simulink library "tramontina_database_nvidialib"  (R2023b)
settings: Solver=VariableStepAuto  StartTime=0.0  StopTime=10.0  RelTol=1e-3
libraries: canmsglib x26, simulink x1
settings Model: Creator=matlab.cut  LastModifiedBy=matlab.cut

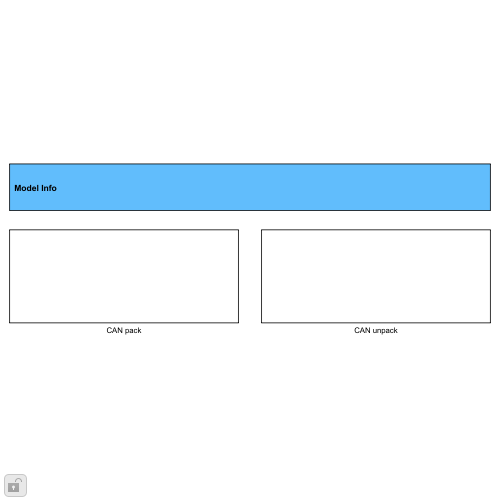
[thumbnail: Simulink's stored preview of the top-level diagram]
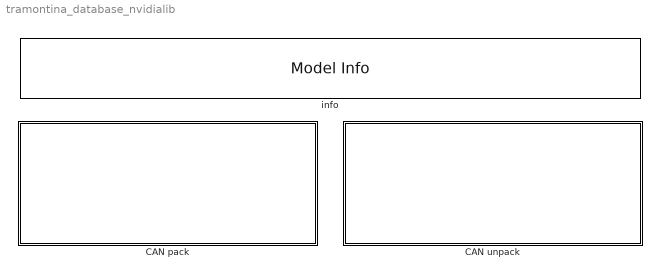
== system tramontina_database_nvidialib ==
  CAN pack : Subsystem
  CAN unpack : Subsystem
  info : simulink/Model-Wide Utilities/Model Info  Frame=on  DisplayStringWithTags=SPEEDGOAT CAN Database Library for: tramontina_database_nvidia  HorizontalTextAlignment=Left  LeftAlignmentValue=0.01

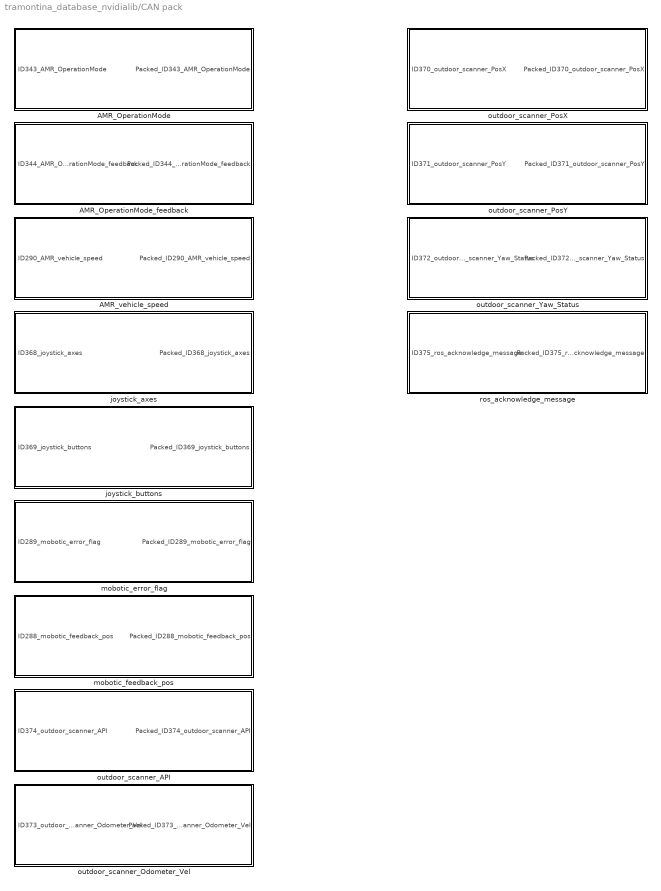
== system tramontina_database_nvidialib/CAN pack ==
  AMR_OperationMode : Subsystem
  AMR_OperationMode_feedback : Subsystem
  AMR_vehicle_speed : Subsystem
  joystick_axes : Subsystem
  joystick_buttons : Subsystem
  mobotic_error_flag : Subsystem
  mobotic_feedback_pos : Subsystem
  outdoor_scanner_API : Subsystem
  outdoor_scanner_Odometer_Vel : Subsystem
  outdoor_scanner_PosX : Subsystem
  outdoor_scanner_PosY : Subsystem
  outdoor_scanner_Yaw_Status : Subsystem
  ros_acknowledge_message : Subsystem

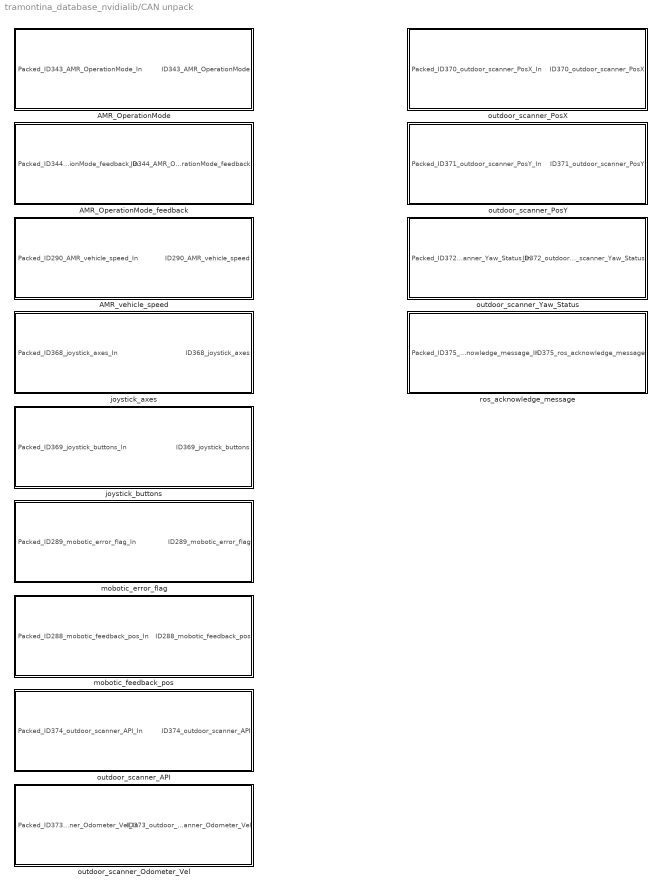
== system tramontina_database_nvidialib/CAN unpack ==
  AMR_OperationMode : Subsystem
  AMR_OperationMode_feedback : Subsystem
  AMR_vehicle_speed : Subsystem
  joystick_axes : Subsystem
  joystick_buttons : Subsystem
  mobotic_error_flag : Subsystem
  mobotic_feedback_pos : Subsystem
  outdoor_scanner_API : Subsystem
  outdoor_scanner_Odometer_Vel : Subsystem
  outdoor_scanner_PosX : Subsystem
  outdoor_scanner_PosY : Subsystem
  outdoor_scanner_Yaw_Status : Subsystem
  ros_acknowledge_message : Subsystem

== system tramontina_database_nvidialib/CAN pack/AMR_OperationMode ==
  In Bus Element : Inport  PortName=ID343_AMR_OperationMode  Element=OperationMode
  AMR_OperationMode : canmsglib/CAN Pack  CANdbFile=C:\Users\matlab.cut\Desktop\AMR\canbus_files\tramontina_database_nvidia.dbc  MsgList=AMR_OperationMode  MsgName=AMR_OperationMode  MsgIDType=Standard (11-bit identifier)  MsgIdentifier=343  MsgLength=8  Remote=off  ApplyMinMax=off  BusOutput=on  SignalInfo={'OperationMode','0','3','LE','unsigned','Standard','0','1','0','-Inf','Inf'}
      settings: DataFormat=manually specified signals
  Packed_ID343_AMR_OperationMode : Outport
  wires:
  AMR_OperationMode/1 -> Packed_ID343_AMR_OperationMode/1
  In Bus Element/1 -> AMR_OperationMode/1

== system tramontina_database_nvidialib/CAN pack/AMR_OperationMode_feedback ==
  In Bus Element : Inport  PortName=ID344_AMR_OperationMode_feedback  Element=OperationMode_auto
  In Bus Element1 : Inport  PortName=ID344_AMR_OperationMode_feedback  Element=OperationMode_idle
  In Bus Element2 : Inport  PortName=ID344_AMR_OperationMode_feedback  Element=OperationMode_manual
  AMR_OperationMode_feedback : canmsglib/CAN Pack  CANdbFile=C:\Users\matlab.cut\Desktop\AMR\canbus_files\tramontina_database_nvidia.dbc  MsgList=AMR_OperationMode_feedback  MsgName=AMR_OperationMode_feedback  MsgIDType=Standard (11-bit identifier)  MsgIdentifier=344  MsgLength=8  Remote=off  ApplyMinMax=off  BusOutput=on  SignalInfo={'OperationMode_auto','2','1','LE','unsigned','Standard','0','1','0','-Inf','Inf';'OperationMode_idle','0','1','LE','unsigned','Standard','0','1','0','-Inf','Inf';'OperationMode_manual','1','1','LE','unsigned','Standard','0','1','0','-Inf','Inf'}
      settings: DataFormat=manually specified signals
  Packed_ID344_AMR_OperationMode_feedback : Outport
  wires:
  AMR_OperationMode_feedback/1 -> Packed_ID344_AMR_OperationMode_feedback/1
  In Bus Element/1 -> AMR_OperationMode_feedback/1
  In Bus Element1/1 -> AMR_OperationMode_feedback/2
  In Bus Element2/1 -> AMR_OperationMode_feedback/3

== system tramontina_database_nvidialib/CAN pack/AMR_vehicle_speed ==
  In Bus Element : Inport  PortName=ID290_AMR_vehicle_speed  Element=speed_m_per_min
  In Bus Element1 : Inport  PortName=ID290_AMR_vehicle_speed  Element=speed_m_per_s
  AMR_vehicle_speed : canmsglib/CAN Pack  CANdbFile=C:\Users\matlab.cut\Desktop\AMR\canbus_files\tramontina_database_nvidia.dbc  MsgList=AMR_vehicle_speed  MsgName=AMR_vehicle_speed  MsgIDType=Standard (11-bit identifier)  MsgIdentifier=290  MsgLength=8  Remote=off  ApplyMinMax=off  BusOutput=on  SignalInfo={'speed_m_per_min','0','32','LE','single','Standard','0','1','0','-90','90';'speed_m_per_s','32','32','LE','single','Standard','0','1','0','-1.5','1.5'}
      settings: DataFormat=manually specified signals
  Packed_ID290_AMR_vehicle_speed : Outport
  wires:
  AMR_vehicle_speed/1 -> Packed_ID290_AMR_vehicle_speed/1
  In Bus Element/1 -> AMR_vehicle_speed/1
  In Bus Element1/1 -> AMR_vehicle_speed/2

== system tramontina_database_nvidialib/CAN pack/joystick_axes ==
  In Bus Element : Inport  PortName=ID368_joystick_axes  Element=joystick_direction
  In Bus Element1 : Inport  PortName=ID368_joystick_axes  Element=joystick_throttle
  joystick_axes : canmsglib/CAN Pack  CANdbFile=C:\Users\matlab.cut\Desktop\AMR\canbus_files\tramontina_database_nvidia.dbc  MsgList=joystick_axes  MsgName=joystick_axes  MsgIDType=Standard (11-bit identifier)  MsgIdentifier=368  MsgLength=8  Remote=off  ApplyMinMax=off  BusOutput=on  SignalInfo={'joystick_direction','56','32','BE','single','Standard','0','1','0','-1','1';'joystick_throttle','24','32','BE','single','Standard','0','1','0','-1','1'}
      settings: DataFormat=manually specified signals
  Packed_ID368_joystick_axes : Outport
  wires:
  joystick_axes/1 -> Packed_ID368_joystick_axes/1
  In Bus Element/1 -> joystick_axes/1
  In Bus Element1/1 -> joystick_axes/2

== system tramontina_database_nvidialib/CAN pack/joystick_buttons ==
  In Bus Element : Inport  PortName=ID369_joystick_buttons  Element=button_5
  In Bus Element1 : Inport  PortName=ID369_joystick_buttons  Element=button_6
  joystick_buttons : canmsglib/CAN Pack  CANdbFile=C:\Users\matlab.cut\Desktop\AMR\canbus_files\tramontina_database_nvidia.dbc  MsgList=joystick_buttons  MsgName=joystick_buttons  MsgIDType=Standard (11-bit identifier)  MsgIdentifier=369  MsgLength=1  Remote=off  ApplyMinMax=off  BusOutput=on  SignalInfo={'button_5','4','1','LE','unsigned','Standard','0','1','0','-Inf','Inf';'button_6','5','1','LE','unsigned','Standard','0','1','0','-Inf','Inf'}
      settings: DataFormat=manually specified signals
  Packed_ID369_joystick_buttons : Outport
  wires:
  joystick_buttons/1 -> Packed_ID369_joystick_buttons/1
  In Bus Element/1 -> joystick_buttons/1
  In Bus Element1/1 -> joystick_buttons/2

== system tramontina_database_nvidialib/CAN pack/mobotic_error_flag ==
  In Bus Element : Inport  PortName=ID289_mobotic_error_flag  Element=steering_unit_error
  mobotic_error_flag : canmsglib/CAN Pack  CANdbFile=C:\Users\matlab.cut\Desktop\AMR\canbus_files\tramontina_database_nvidia.dbc  MsgList=mobotic_error_flag  MsgName=mobotic_error_flag  MsgIDType=Standard (11-bit identifier)  MsgIdentifier=289  MsgLength=8  Remote=off  ApplyMinMax=off  BusOutput=on  SignalInfo={'steering_unit_error','0','1','LE','unsigned','Standard','0','1','0','-Inf','Inf'}
      settings: DataFormat=manually specified signals
  Packed_ID289_mobotic_error_flag : Outport
  wires:
  mobotic_error_flag/1 -> Packed_ID289_mobotic_error_flag/1
  In Bus Element/1 -> mobotic_error_flag/1

== system tramontina_database_nvidialib/CAN pack/mobotic_feedback_pos ==
  In Bus Element : Inport  PortName=ID288_mobotic_feedback_pos  Element=enconder_feedback
  In Bus Element1 : Inport  PortName=ID288_mobotic_feedback_pos  Element=position_feedback
  mobotic_feedback_pos : canmsglib/CAN Pack  CANdbFile=C:\Users\matlab.cut\Desktop\AMR\canbus_files\tramontina_database_nvidia.dbc  MsgList=mobotic_feedback_pos  MsgName=mobotic_feedback_pos  MsgIDType=Standard (11-bit identifier)  MsgIdentifier=288  MsgLength=8  Remote=off  ApplyMinMax=off  BusOutput=on  SignalInfo={'enconder_feedback','32','32','LE','signed','Standard','0','1','0','-Inf','Inf';'position_feedback','0','32','LE','signed','Standard','0','0.087891','30','-75','75'}
      settings: DataFormat=manually specified signals
  Packed_ID288_mobotic_feedback_pos : Outport
  wires:
  mobotic_feedback_pos/1 -> Packed_ID288_mobotic_feedback_pos/1
  In Bus Element/1 -> mobotic_feedback_pos/1
  In Bus Element1/1 -> mobotic_feedback_pos/2

== system tramontina_database_nvidialib/CAN pack/outdoor_scanner_API ==
  In Bus Element : Inport  PortName=ID374_outdoor_scanner_API  Element=LocClearMap
  In Bus Element1 : Inport  PortName=ID374_outdoor_scanner_API  Element=LocInitAtPose
  In Bus Element2 : Inport  PortName=ID374_outdoor_scanner_API  Element=LocLoadMap
  In Bus Element3 : Inport  PortName=ID374_outdoor_scanner_API  Element=LocSetMap
  In Bus Element4 : Inport  PortName=ID374_outdoor_scanner_API  Element=MapID
  outdoor_scanner_API : canmsglib/CAN Pack  CANdbFile=C:\Users\matlab.cut\Desktop\AMR\canbus_files\tramontina_database_nvidia.dbc  MsgList=outdoor_scanner_API  MsgName=outdoor_scanner_API  MsgIDType=Standard (11-bit identifier)  MsgIdentifier=374  MsgLength=2  Remote=off  ApplyMinMax=off  BusOutput=on  SignalInfo={'LocClearMap','10','1','LE','unsigned','Standard','0','1','0','0','1';'LocInitAtPose','11','1','LE','unsigned','Standard','0','1','0','0','1';'LocLoadMap','9','1','LE','unsigned','Standard','0','1','0','0','1';'LocSetMap','8','1','LE','unsigned','Standard','0','1','0','0','1';'MapID','0','8','LE','unsigned','Standard','0','1','0','-Inf','Inf'}
      settings: DataFormat=manually specified signals
  Packed_ID374_outdoor_scanner_API : Outport
  wires:
  outdoor_scanner_API/1 -> Packed_ID374_outdoor_scanner_API/1
  In Bus Element/1 -> outdoor_scanner_API/1
  In Bus Element1/1 -> outdoor_scanner_API/2
  In Bus Element2/1 -> outdoor_scanner_API/3
  In Bus Element3/1 -> outdoor_scanner_API/4
  In Bus Element4/1 -> outdoor_scanner_API/5

== system tramontina_database_nvidialib/CAN pack/outdoor_scanner_Odometer_Vel ==
  In Bus Element : Inport  PortName=ID373_outdoor_scanner_Odometer_Vel  Element=velAng
  In Bus Element1 : Inport  PortName=ID373_outdoor_scanner_Odometer_Vel  Element=velX
  In Bus Element2 : Inport  PortName=ID373_outdoor_scanner_Odometer_Vel  Element=velY
  outdoor_scanner_Odometer_Vel : canmsglib/CAN Pack  CANdbFile=C:\Users\matlab.cut\Desktop\AMR\canbus_files\tramontina_database_nvidia.dbc  MsgList=outdoor_scanner_Odometer_Vel  MsgName=outdoor_scanner_Odometer_Vel  MsgIDType=Standard (11-bit identifier)  MsgIdentifier=373  MsgLength=8  Remote=off  ApplyMinMax=off  BusOutput=on  SignalInfo={'velAng','32','32','LE','single','Standard','0','1','0','-2147483648','-2147483648';'velX','0','16','LE','signed','Standard','0','1','0','-32768','32768';'velY','16','16','LE','signed','Standard','0','1','0','-32768','32768'}
      settings: DataFormat=manually specified signals
  Packed_ID373_outdoor_scanner_Odometer_Vel : Outport
  wires:
  outdoor_scanner_Odometer_Vel/1 -> Packed_ID373_outdoor_scanner_Odometer_Vel/1
  In Bus Element/1 -> outdoor_scanner_Odometer_Vel/1
  In Bus Element1/1 -> outdoor_scanner_Odometer_Vel/2
  In Bus Element2/1 -> outdoor_scanner_Odometer_Vel/3

== system tramontina_database_nvidialib/CAN pack/outdoor_scanner_PosX ==
  In Bus Element : Inport  PortName=ID370_outdoor_scanner_PosX  Element=X
  outdoor_scanner_PosX : canmsglib/CAN Pack  CANdbFile=C:\Users\matlab.cut\Desktop\AMR\canbus_files\tramontina_database_nvidia.dbc  MsgList=outdoor_scanner_PosX  MsgName=outdoor_scanner_PosX  MsgIDType=Standard (11-bit identifier)  MsgIdentifier=370  MsgLength=8  Remote=off  ApplyMinMax=off  BusOutput=on  SignalInfo={'X','0','64','LE','double','Standard','0','1','0','-9.2233720369e+18','9.2233720369e+18'}
      settings: DataFormat=manually specified signals
  Packed_ID370_outdoor_scanner_PosX : Outport
  wires:
  outdoor_scanner_PosX/1 -> Packed_ID370_outdoor_scanner_PosX/1
  In Bus Element/1 -> outdoor_scanner_PosX/1

== system tramontina_database_nvidialib/CAN pack/outdoor_scanner_PosY ==
  In Bus Element : Inport  PortName=ID371_outdoor_scanner_PosY  Element=Y
  outdoor_scanner_PosY : canmsglib/CAN Pack  CANdbFile=C:\Users\matlab.cut\Desktop\AMR\canbus_files\tramontina_database_nvidia.dbc  MsgList=outdoor_scanner_PosY  MsgName=outdoor_scanner_PosY  MsgIDType=Standard (11-bit identifier)  MsgIdentifier=371  MsgLength=8  Remote=off  ApplyMinMax=off  BusOutput=on  SignalInfo={'Y','0','64','LE','double','Standard','0','1','0','-9.2233720369e+18','9.2233720369e+18'}
      settings: DataFormat=manually specified signals
  Packed_ID371_outdoor_scanner_PosY : Outport
  wires:
  outdoor_scanner_PosY/1 -> Packed_ID371_outdoor_scanner_PosY/1
  In Bus Element/1 -> outdoor_scanner_PosY/1

== system tramontina_database_nvidialib/CAN pack/outdoor_scanner_Yaw_Status ==
  In Bus Element : Inport  PortName=ID372_outdoor_scanner_Yaw_Status  Element=LocalizationStatus
  In Bus Element1 : Inport  PortName=ID372_outdoor_scanner_Yaw_Status  Element=MapMatchingStatus
  In Bus Element2 : Inport  PortName=ID372_outdoor_scanner_Yaw_Status  Element=Yaw
  outdoor_scanner_Yaw_Status : canmsglib/CAN Pack  CANdbFile=C:\Users\matlab.cut\Desktop\AMR\canbus_files\tramontina_database_nvidia.dbc  MsgList=outdoor_scanner_Yaw_Status  MsgName=outdoor_scanner_Yaw_Status  MsgIDType=Standard (11-bit identifier)  MsgIdentifier=372  MsgLength=6  Remote=off  ApplyMinMax=off  BusOutput=on  SignalInfo={'LocalizationStatus','32','8','LE','unsigned','Standard','0','1','0','-Inf','Inf';'MapMatchingStatus','40','8','LE','unsigned','Standard','0','1','0','-Inf','Inf';'Yaw','0','32','LE','signed','Standard','0','1','0','-180000','180000'}
      settings: DataFormat=manually specified signals
  Packed_ID372_outdoor_scanner_Yaw_Status : Outport
  wires:
  outdoor_scanner_Yaw_Status/1 -> Packed_ID372_outdoor_scanner_Yaw_Status/1
  In Bus Element/1 -> outdoor_scanner_Yaw_Status/1
  In Bus Element1/1 -> outdoor_scanner_Yaw_Status/2
  In Bus Element2/1 -> outdoor_scanner_Yaw_Status/3

== system tramontina_database_nvidialib/CAN pack/ros_acknowledge_message ==
  In Bus Element : Inport  PortName=ID375_ros_acknowledge_message  Element=ack_LocInitAtPose
  In Bus Element1 : Inport  PortName=ID375_ros_acknowledge_message  Element=ack_LocSetMap
  In Bus Element2 : Inport  PortName=ID375_ros_acknowledge_message  Element=ack_NewMapName_received
  In Bus Element3 : Inport  PortName=ID375_ros_acknowledge_message  Element=ack_NewPose_received
  In Bus Element4 : Inport  PortName=ID375_ros_acknowledge_message  Element=ack_id_received
  ros_acknowledge_message : canmsglib/CAN Pack  CANdbFile=C:\Users\matlab.cut\Desktop\AMR\canbus_files\tramontina_database_nvidia.dbc  MsgList=ros_acknowledge_message  MsgName=ros_acknowledge_message  MsgIDType=Standard (11-bit identifier)  MsgIdentifier=375  MsgLength=1  Remote=off  ApplyMinMax=off  BusOutput=on  SignalInfo={'ack_LocInitAtPose','3','1','LE','unsigned','Standard','0','1','0','-Inf','Inf';'ack_LocSetMap','4','1','LE','unsigned','Standard','0','1','0','-Inf','Inf';'ack_NewMapName_received','1','1','LE','unsigned','Standard','0','1','0','-Inf','Inf';'ack_NewPose_received','2','1','LE','unsigned','Standard','0','1','0','-Inf','Inf';'ack_id_received','0','1','LE','unsigned','Standard','0','1','0','0','1'}
      settings: DataFormat=manually specified signals
  Packed_ID375_ros_acknowledge_message : Outport
  wires:
  ros_acknowledge_message/1 -> Packed_ID375_ros_acknowledge_message/1
  In Bus Element/1 -> ros_acknowledge_message/1
  In Bus Element1/1 -> ros_acknowledge_message/2
  In Bus Element2/1 -> ros_acknowledge_message/3
  In Bus Element3/1 -> ros_acknowledge_message/4
  In Bus Element4/1 -> ros_acknowledge_message/5

== system tramontina_database_nvidialib/CAN unpack/AMR_OperationMode ==
  Packed_ID343_AMR_OperationMode_In : Inport
  AMR_OperationMode : canmsglib/CAN Unpack  CANdbFile=C:\Users\matlab.cut\Desktop\AMR\canbus_files\tramontina_database_nvidia.dbc  MsgList=AMR_OperationMode  MsgName=AMR_OperationMode  MsgIDType=Standard (11-bit identifier)  MsgIdentifier=343  MsgLength=8  SignalInfo={'OperationMode','0','3','LE','unsigned','Standard','0','1','0','-Inf','Inf'}  IDPort=on  TimestampPort=on  ErrorPort=on  RemotePort=on  LengthPort=on  StatusPort=on  ApplyMinMax=off
  Out Bus Element : Outport  PortName=ID343_AMR_OperationMode  Element=OperationMode
  Out Bus Element1 : Outport  PortName=ID343_AMR_OperationMode  Element=MessageStatus.ID
  Out Bus Element2 : Outport  PortName=ID343_AMR_OperationMode  Element=MessageStatus.Timestamp
  Out Bus Element3 : Outport  PortName=ID343_AMR_OperationMode  Element=MessageStatus.Error
  Out Bus Element4 : Outport  PortName=ID343_AMR_OperationMode  Element=MessageStatus.Remote
  Out Bus Element5 : Outport  PortName=ID343_AMR_OperationMode  Element=MessageStatus.Length
  Out Bus Element6 : Outport  PortName=ID343_AMR_OperationMode  Element=MessageStatus.Status
  wires:
  Packed_ID343_AMR_OperationMode_In/1 -> AMR_OperationMode/1
  AMR_OperationMode/1 -> Out Bus Element/1  "ID343_AMR_OperationMode.OperationMode"
  AMR_OperationMode/2 -> Out Bus Element1/1  "ID343_AMR_OperationMode.MessageStatus.ID"
  AMR_OperationMode/3 -> Out Bus Element2/1  "ID343_AMR_OperationMode.MessageStatus.Timestamp"
  AMR_OperationMode/4 -> Out Bus Element3/1  "ID343_AMR_OperationMode.MessageStatus.Error"
  AMR_OperationMode/5 -> Out Bus Element4/1  "ID343_AMR_OperationMode.MessageStatus.Remote"
  AMR_OperationMode/6 -> Out Bus Element5/1  "ID343_AMR_OperationMode.MessageStatus.Length"
  AMR_OperationMode/7 -> Out Bus Element6/1  "ID343_AMR_OperationMode.MessageStatus.Status"

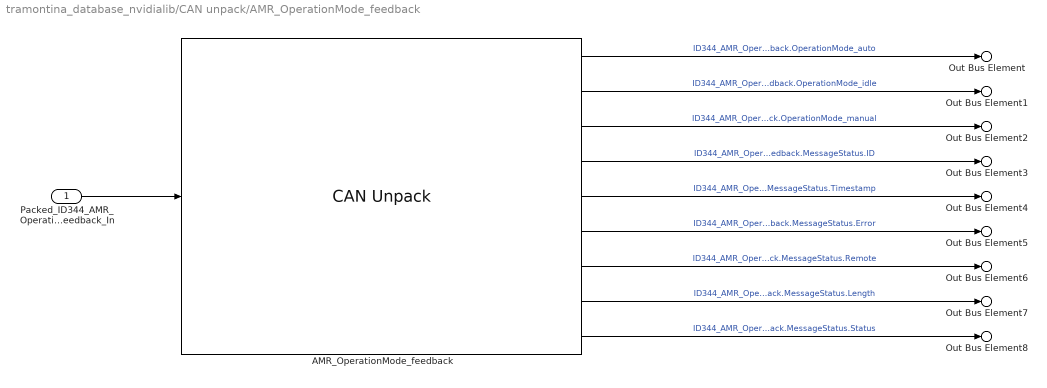
== system tramontina_database_nvidialib/CAN unpack/AMR_OperationMode_feedback ==
  Packed_ID344_AMR_OperationMode_feedback_In : Inport
  AMR_OperationMode_feedback : canmsglib/CAN Unpack  CANdbFile=C:\Users\matlab.cut\Desktop\AMR\canbus_files\tramontina_database_nvidia.dbc  MsgList=AMR_OperationMode_feedback  MsgName=AMR_OperationMode_feedback  MsgIDType=Standard (11-bit identifier)  MsgIdentifier=344  MsgLength=8  SignalInfo={'OperationMode_auto','2','1','LE','unsigned','Standard','0','1','0','-Inf','Inf';'OperationMode_idle','0','1','LE','unsigned','Standard','0','1','0','-Inf','Inf';'OperationMode_manual','1','1','LE','unsigned','Standard','0','1','0','-Inf','Inf'}  IDPort=on  TimestampPort=on  ErrorPort=on  RemotePort=on  LengthPort=on  StatusPort=on  ApplyMinMax=off
  Out Bus Element : Outport  PortName=ID344_AMR_OperationMode_feedback  Element=OperationMode_auto
  Out Bus Element1 : Outport  PortName=ID344_AMR_OperationMode_feedback  Element=OperationMode_idle
  Out Bus Element2 : Outport  PortName=ID344_AMR_OperationMode_feedback  Element=OperationMode_manual
  Out Bus Element3 : Outport  PortName=ID344_AMR_OperationMode_feedback  Element=MessageStatus.ID
  Out Bus Element4 : Outport  PortName=ID344_AMR_OperationMode_feedback  Element=MessageStatus.Timestamp
  Out Bus Element5 : Outport  PortName=ID344_AMR_OperationMode_feedback  Element=MessageStatus.Error
  Out Bus Element6 : Outport  PortName=ID344_AMR_OperationMode_feedback  Element=MessageStatus.Remote
  Out Bus Element7 : Outport  PortName=ID344_AMR_OperationMode_feedback  Element=MessageStatus.Length
  Out Bus Element8 : Outport  PortName=ID344_AMR_OperationMode_feedback  Element=MessageStatus.Status
  wires:
  Packed_ID344_AMR_OperationMode_feedback_In/1 -> AMR_OperationMode_feedback/1
  AMR_OperationMode_feedback/1 -> Out Bus Element/1  "ID344_AMR_OperationMode_feedback.OperationMode_auto"
  AMR_OperationMode_feedback/2 -> Out Bus Element1/1  "ID344_AMR_OperationMode_feedback.OperationMode_idle"
  AMR_OperationMode_feedback/3 -> Out Bus Element2/1  "ID344_AMR_OperationMode_feedback.OperationMode_manual"
  AMR_OperationMode_feedback/4 -> Out Bus Element3/1  "ID344_AMR_OperationMode_feedback.MessageStatus.ID"
  AMR_OperationMode_feedback/5 -> Out Bus Element4/1  "ID344_AMR_OperationMode_feedback.MessageStatus.Timestamp"
  AMR_OperationMode_feedback/6 -> Out Bus Element5/1  "ID344_AMR_OperationMode_feedback.MessageStatus.Error"
  AMR_OperationMode_feedback/7 -> Out Bus Element6/1  "ID344_AMR_OperationMode_feedback.MessageStatus.Remote"
  AMR_OperationMode_feedback/8 -> Out Bus Element7/1  "ID344_AMR_OperationMode_feedback.MessageStatus.Length"
  AMR_OperationMode_feedback/9 -> Out Bus Element8/1  "ID344_AMR_OperationMode_feedback.MessageStatus.Status"

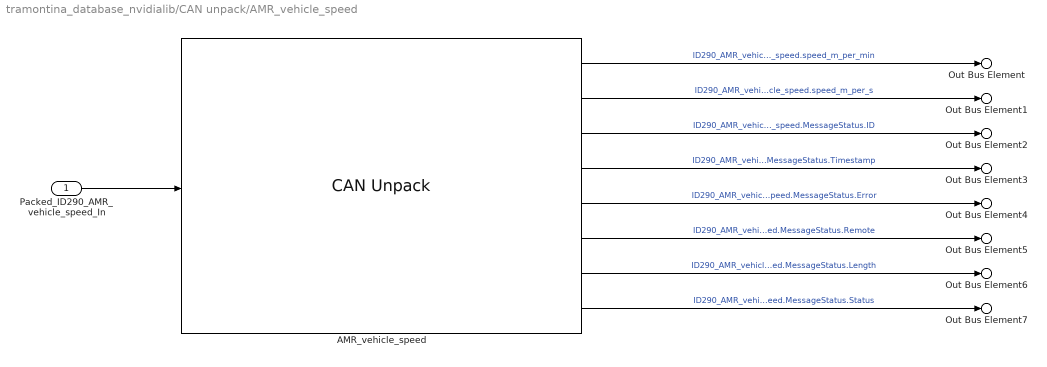
== system tramontina_database_nvidialib/CAN unpack/AMR_vehicle_speed ==
  Packed_ID290_AMR_vehicle_speed_In : Inport
  AMR_vehicle_speed : canmsglib/CAN Unpack  CANdbFile=C:\Users\matlab.cut\Desktop\AMR\canbus_files\tramontina_database_nvidia.dbc  MsgList=AMR_vehicle_speed  MsgName=AMR_vehicle_speed  MsgIDType=Standard (11-bit identifier)  MsgIdentifier=290  MsgLength=8  SignalInfo={'speed_m_per_min','0','32','LE','single','Standard','0','1','0','-90','90';'speed_m_per_s','32','32','LE','single','Standard','0','1','0','-1.5','1.5'}  IDPort=on  TimestampPort=on  ErrorPort=on  RemotePort=on  LengthPort=on  StatusPort=on  ApplyMinMax=off
  Out Bus Element : Outport  PortName=ID290_AMR_vehicle_speed  Element=speed_m_per_min
  Out Bus Element1 : Outport  PortName=ID290_AMR_vehicle_speed  Element=speed_m_per_s
  Out Bus Element2 : Outport  PortName=ID290_AMR_vehicle_speed  Element=MessageStatus.ID
  Out Bus Element3 : Outport  PortName=ID290_AMR_vehicle_speed  Element=MessageStatus.Timestamp
  Out Bus Element4 : Outport  PortName=ID290_AMR_vehicle_speed  Element=MessageStatus.Error
  Out Bus Element5 : Outport  PortName=ID290_AMR_vehicle_speed  Element=MessageStatus.Remote
  Out Bus Element6 : Outport  PortName=ID290_AMR_vehicle_speed  Element=MessageStatus.Length
  Out Bus Element7 : Outport  PortName=ID290_AMR_vehicle_speed  Element=MessageStatus.Status
  wires:
  Packed_ID290_AMR_vehicle_speed_In/1 -> AMR_vehicle_speed/1
  AMR_vehicle_speed/1 -> Out Bus Element/1  "ID290_AMR_vehicle_speed.speed_m_per_min"
  AMR_vehicle_speed/2 -> Out Bus Element1/1  "ID290_AMR_vehicle_speed.speed_m_per_s"
  AMR_vehicle_speed/3 -> Out Bus Element2/1  "ID290_AMR_vehicle_speed.MessageStatus.ID"
  AMR_vehicle_speed/4 -> Out Bus Element3/1  "ID290_AMR_vehicle_speed.MessageStatus.Timestamp"
  AMR_vehicle_speed/5 -> Out Bus Element4/1  "ID290_AMR_vehicle_speed.MessageStatus.Error"
  AMR_vehicle_speed/6 -> Out Bus Element5/1  "ID290_AMR_vehicle_speed.MessageStatus.Remote"
  AMR_vehicle_speed/7 -> Out Bus Element6/1  "ID290_AMR_vehicle_speed.MessageStatus.Length"
  AMR_vehicle_speed/8 -> Out Bus Element7/1  "ID290_AMR_vehicle_speed.MessageStatus.Status"

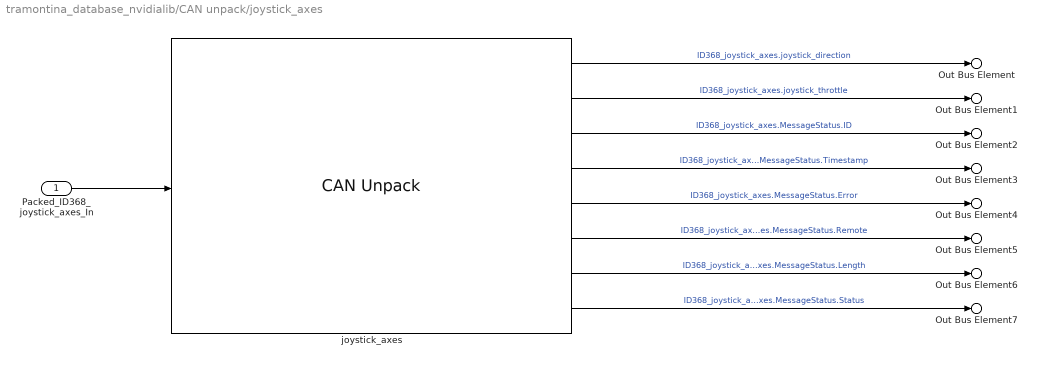
== system tramontina_database_nvidialib/CAN unpack/joystick_axes ==
  Packed_ID368_joystick_axes_In : Inport
  joystick_axes : canmsglib/CAN Unpack  CANdbFile=C:\Users\matlab.cut\Desktop\AMR\canbus_files\tramontina_database_nvidia.dbc  MsgList=joystick_axes  MsgName=joystick_axes  MsgIDType=Standard (11-bit identifier)  MsgIdentifier=368  MsgLength=8  SignalInfo={'joystick_direction','56','32','BE','single','Standard','0','1','0','-1','1';'joystick_throttle','24','32','BE','single','Standard','0','1','0','-1','1'}  IDPort=on  TimestampPort=on  ErrorPort=on  RemotePort=on  LengthPort=on  StatusPort=on  ApplyMinMax=off
  Out Bus Element : Outport  PortName=ID368_joystick_axes  Element=joystick_direction
  Out Bus Element1 : Outport  PortName=ID368_joystick_axes  Element=joystick_throttle
  Out Bus Element2 : Outport  PortName=ID368_joystick_axes  Element=MessageStatus.ID
  Out Bus Element3 : Outport  PortName=ID368_joystick_axes  Element=MessageStatus.Timestamp
  Out Bus Element4 : Outport  PortName=ID368_joystick_axes  Element=MessageStatus.Error
  Out Bus Element5 : Outport  PortName=ID368_joystick_axes  Element=MessageStatus.Remote
  Out Bus Element6 : Outport  PortName=ID368_joystick_axes  Element=MessageStatus.Length
  Out Bus Element7 : Outport  PortName=ID368_joystick_axes  Element=MessageStatus.Status
  wires:
  Packed_ID368_joystick_axes_In/1 -> joystick_axes/1
  joystick_axes/1 -> Out Bus Element/1  "ID368_joystick_axes.joystick_direction"
  joystick_axes/2 -> Out Bus Element1/1  "ID368_joystick_axes.joystick_throttle"
  joystick_axes/3 -> Out Bus Element2/1  "ID368_joystick_axes.MessageStatus.ID"
  joystick_axes/4 -> Out Bus Element3/1  "ID368_joystick_axes.MessageStatus.Timestamp"
  joystick_axes/5 -> Out Bus Element4/1  "ID368_joystick_axes.MessageStatus.Error"
  joystick_axes/6 -> Out Bus Element5/1  "ID368_joystick_axes.MessageStatus.Remote"
  joystick_axes/7 -> Out Bus Element6/1  "ID368_joystick_axes.MessageStatus.Length"
  joystick_axes/8 -> Out Bus Element7/1  "ID368_joystick_axes.MessageStatus.Status"

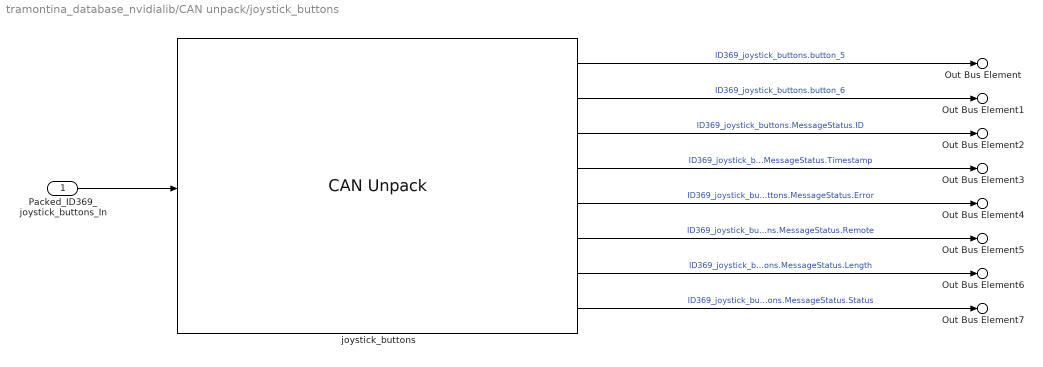
== system tramontina_database_nvidialib/CAN unpack/joystick_buttons ==
  Packed_ID369_joystick_buttons_In : Inport
  joystick_buttons : canmsglib/CAN Unpack  CANdbFile=C:\Users\matlab.cut\Desktop\AMR\canbus_files\tramontina_database_nvidia.dbc  MsgList=joystick_buttons  MsgName=joystick_buttons  MsgIDType=Standard (11-bit identifier)  MsgIdentifier=369  MsgLength=1  SignalInfo={'button_5','4','1','LE','unsigned','Standard','0','1','0','-Inf','Inf';'button_6','5','1','LE','unsigned','Standard','0','1','0','-Inf','Inf'}  IDPort=on  TimestampPort=on  ErrorPort=on  RemotePort=on  LengthPort=on  StatusPort=on  ApplyMinMax=off
  Out Bus Element : Outport  PortName=ID369_joystick_buttons  Element=button_5
  Out Bus Element1 : Outport  PortName=ID369_joystick_buttons  Element=button_6
  Out Bus Element2 : Outport  PortName=ID369_joystick_buttons  Element=MessageStatus.ID
  Out Bus Element3 : Outport  PortName=ID369_joystick_buttons  Element=MessageStatus.Timestamp
  Out Bus Element4 : Outport  PortName=ID369_joystick_buttons  Element=MessageStatus.Error
  Out Bus Element5 : Outport  PortName=ID369_joystick_buttons  Element=MessageStatus.Remote
  Out Bus Element6 : Outport  PortName=ID369_joystick_buttons  Element=MessageStatus.Length
  Out Bus Element7 : Outport  PortName=ID369_joystick_buttons  Element=MessageStatus.Status
  wires:
  Packed_ID369_joystick_buttons_In/1 -> joystick_buttons/1
  joystick_buttons/1 -> Out Bus Element/1  "ID369_joystick_buttons.button_5"
  joystick_buttons/2 -> Out Bus Element1/1  "ID369_joystick_buttons.button_6"
  joystick_buttons/3 -> Out Bus Element2/1  "ID369_joystick_buttons.MessageStatus.ID"
  joystick_buttons/4 -> Out Bus Element3/1  "ID369_joystick_buttons.MessageStatus.Timestamp"
  joystick_buttons/5 -> Out Bus Element4/1  "ID369_joystick_buttons.MessageStatus.Error"
  joystick_buttons/6 -> Out Bus Element5/1  "ID369_joystick_buttons.MessageStatus.Remote"
  joystick_buttons/7 -> Out Bus Element6/1  "ID369_joystick_buttons.MessageStatus.Length"
  joystick_buttons/8 -> Out Bus Element7/1  "ID369_joystick_buttons.MessageStatus.Status"

== system tramontina_database_nvidialib/CAN unpack/mobotic_error_flag ==
  Packed_ID289_mobotic_error_flag_In : Inport
  mobotic_error_flag : canmsglib/CAN Unpack  CANdbFile=C:\Users\matlab.cut\Desktop\AMR\canbus_files\tramontina_database_nvidia.dbc  MsgList=mobotic_error_flag  MsgName=mobotic_error_flag  MsgIDType=Standard (11-bit identifier)  MsgIdentifier=289  MsgLength=8  SignalInfo={'steering_unit_error','0','1','LE','unsigned','Standard','0','1','0','-Inf','Inf'}  IDPort=on  TimestampPort=on  ErrorPort=on  RemotePort=on  LengthPort=on  StatusPort=on  ApplyMinMax=off
  Out Bus Element : Outport  PortName=ID289_mobotic_error_flag  Element=steering_unit_error
  Out Bus Element1 : Outport  PortName=ID289_mobotic_error_flag  Element=MessageStatus.ID
  Out Bus Element2 : Outport  PortName=ID289_mobotic_error_flag  Element=MessageStatus.Timestamp
  Out Bus Element3 : Outport  PortName=ID289_mobotic_error_flag  Element=MessageStatus.Error
  Out Bus Element4 : Outport  PortName=ID289_mobotic_error_flag  Element=MessageStatus.Remote
  Out Bus Element5 : Outport  PortName=ID289_mobotic_error_flag  Element=MessageStatus.Length
  Out Bus Element6 : Outport  PortName=ID289_mobotic_error_flag  Element=MessageStatus.Status
  wires:
  Packed_ID289_mobotic_error_flag_In/1 -> mobotic_error_flag/1
  mobotic_error_flag/1 -> Out Bus Element/1  "ID289_mobotic_error_flag.steering_unit_error"
  mobotic_error_flag/2 -> Out Bus Element1/1  "ID289_mobotic_error_flag.MessageStatus.ID"
  mobotic_error_flag/3 -> Out Bus Element2/1  "ID289_mobotic_error_flag.MessageStatus.Timestamp"
  mobotic_error_flag/4 -> Out Bus Element3/1  "ID289_mobotic_error_flag.MessageStatus.Error"
  mobotic_error_flag/5 -> Out Bus Element4/1  "ID289_mobotic_error_flag.MessageStatus.Remote"
  mobotic_error_flag/6 -> Out Bus Element5/1  "ID289_mobotic_error_flag.MessageStatus.Length"
  mobotic_error_flag/7 -> Out Bus Element6/1  "ID289_mobotic_error_flag.MessageStatus.Status"

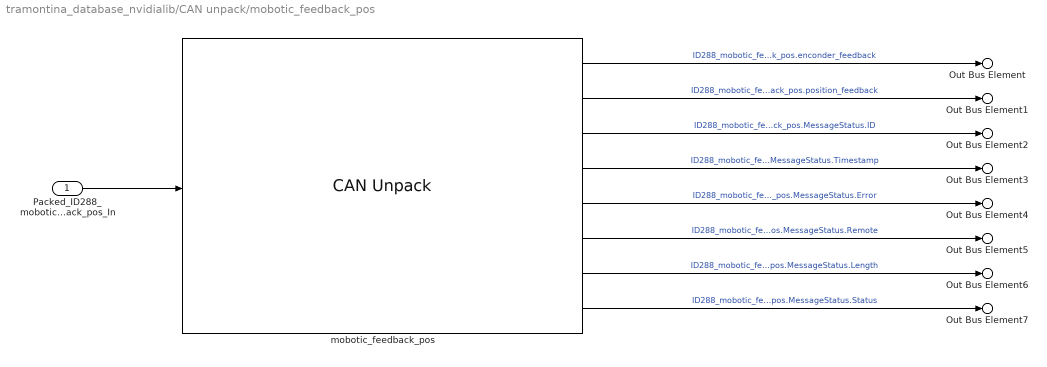
== system tramontina_database_nvidialib/CAN unpack/mobotic_feedback_pos ==
  Packed_ID288_mobotic_feedback_pos_In : Inport
  mobotic_feedback_pos : canmsglib/CAN Unpack  CANdbFile=C:\Users\matlab.cut\Desktop\AMR\canbus_files\tramontina_database_nvidia.dbc  MsgList=mobotic_feedback_pos  MsgName=mobotic_feedback_pos  MsgIDType=Standard (11-bit identifier)  MsgIdentifier=288  MsgLength=8  SignalInfo={'enconder_feedback','32','32','LE','signed','Standard','0','1','0','-Inf','Inf';'position_feedback','0','32','LE','signed','Standard','0','0.087891','30','-75','75'}  IDPort=on  TimestampPort=on  ErrorPort=on  RemotePort=on  LengthPort=on  StatusPort=on  ApplyMinMax=off
  Out Bus Element : Outport  PortName=ID288_mobotic_feedback_pos  Element=enconder_feedback
  Out Bus Element1 : Outport  PortName=ID288_mobotic_feedback_pos  Element=position_feedback
  Out Bus Element2 : Outport  PortName=ID288_mobotic_feedback_pos  Element=MessageStatus.ID
  Out Bus Element3 : Outport  PortName=ID288_mobotic_feedback_pos  Element=MessageStatus.Timestamp
  Out Bus Element4 : Outport  PortName=ID288_mobotic_feedback_pos  Element=MessageStatus.Error
  Out Bus Element5 : Outport  PortName=ID288_mobotic_feedback_pos  Element=MessageStatus.Remote
  Out Bus Element6 : Outport  PortName=ID288_mobotic_feedback_pos  Element=MessageStatus.Length
  Out Bus Element7 : Outport  PortName=ID288_mobotic_feedback_pos  Element=MessageStatus.Status
  wires:
  Packed_ID288_mobotic_feedback_pos_In/1 -> mobotic_feedback_pos/1
  mobotic_feedback_pos/1 -> Out Bus Element/1  "ID288_mobotic_feedback_pos.enconder_feedback"
  mobotic_feedback_pos/2 -> Out Bus Element1/1  "ID288_mobotic_feedback_pos.position_feedback"
  mobotic_feedback_pos/3 -> Out Bus Element2/1  "ID288_mobotic_feedback_pos.MessageStatus.ID"
  mobotic_feedback_pos/4 -> Out Bus Element3/1  "ID288_mobotic_feedback_pos.MessageStatus.Timestamp"
  mobotic_feedback_pos/5 -> Out Bus Element4/1  "ID288_mobotic_feedback_pos.MessageStatus.Error"
  mobotic_feedback_pos/6 -> Out Bus Element5/1  "ID288_mobotic_feedback_pos.MessageStatus.Remote"
  mobotic_feedback_pos/7 -> Out Bus Element6/1  "ID288_mobotic_feedback_pos.MessageStatus.Length"
  mobotic_feedback_pos/8 -> Out Bus Element7/1  "ID288_mobotic_feedback_pos.MessageStatus.Status"

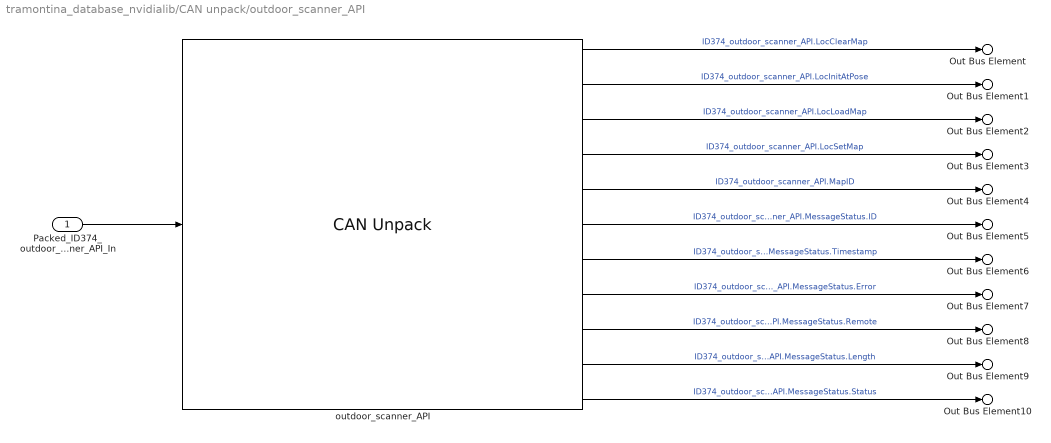
== system tramontina_database_nvidialib/CAN unpack/outdoor_scanner_API ==
  Packed_ID374_outdoor_scanner_API_In : Inport
  outdoor_scanner_API : canmsglib/CAN Unpack  CANdbFile=C:\Users\matlab.cut\Desktop\AMR\canbus_files\tramontina_database_nvidia.dbc  MsgList=outdoor_scanner_API  MsgName=outdoor_scanner_API  MsgIDType=Standard (11-bit identifier)  MsgIdentifier=374  MsgLength=2  SignalInfo={'LocClearMap','10','1','LE','unsigned','Standard','0','1','0','0','1';'LocInitAtPose','11','1','LE','unsigned','Standard','0','1','0','0','1';'LocLoadMap','9','1','LE','unsigned','Standard','0','1','0','0','1';'LocSetMap','8','1','LE','unsigned','Standard','0','1','0','0','1';'MapID','0','8','LE','unsigned','Standard','0','1','0','-Inf','Inf'}  IDPort=on  TimestampPort=on  ErrorPort=on  RemotePort=on  LengthPort=on  StatusPort=on  ApplyMinMax=off
  Out Bus Element : Outport  PortName=ID374_outdoor_scanner_API  Element=LocClearMap
  Out Bus Element1 : Outport  PortName=ID374_outdoor_scanner_API  Element=LocInitAtPose
  Out Bus Element2 : Outport  PortName=ID374_outdoor_scanner_API  Element=LocLoadMap
  Out Bus Element3 : Outport  PortName=ID374_outdoor_scanner_API  Element=LocSetMap
  Out Bus Element4 : Outport  PortName=ID374_outdoor_scanner_API  Element=MapID
  Out Bus Element5 : Outport  PortName=ID374_outdoor_scanner_API  Element=MessageStatus.ID
  Out Bus Element6 : Outport  PortName=ID374_outdoor_scanner_API  Element=MessageStatus.Timestamp
  Out Bus Element7 : Outport  PortName=ID374_outdoor_scanner_API  Element=MessageStatus.Error
  Out Bus Element8 : Outport  PortName=ID374_outdoor_scanner_API  Element=MessageStatus.Remote
  Out Bus Element9 : Outport  PortName=ID374_outdoor_scanner_API  Element=MessageStatus.Length
  Out Bus Element10 : Outport  PortName=ID374_outdoor_scanner_API  Element=MessageStatus.Status
  wires:
  Packed_ID374_outdoor_scanner_API_In/1 -> outdoor_scanner_API/1
  outdoor_scanner_API/1 -> Out Bus Element/1  "ID374_outdoor_scanner_API.LocClearMap"
  outdoor_scanner_API/2 -> Out Bus Element1/1  "ID374_outdoor_scanner_API.LocInitAtPose"
  outdoor_scanner_API/3 -> Out Bus Element2/1  "ID374_outdoor_scanner_API.LocLoadMap"
  outdoor_scanner_API/4 -> Out Bus Element3/1  "ID374_outdoor_scanner_API.LocSetMap"
  outdoor_scanner_API/5 -> Out Bus Element4/1  "ID374_outdoor_scanner_API.MapID"
  outdoor_scanner_API/6 -> Out Bus Element5/1  "ID374_outdoor_scanner_API.MessageStatus.ID"
  outdoor_scanner_API/7 -> Out Bus Element6/1  "ID374_outdoor_scanner_API.MessageStatus.Timestamp"
  outdoor_scanner_API/8 -> Out Bus Element7/1  "ID374_outdoor_scanner_API.MessageStatus.Error"
  outdoor_scanner_API/9 -> Out Bus Element8/1  "ID374_outdoor_scanner_API.MessageStatus.Remote"
  outdoor_scanner_API/10 -> Out Bus Element9/1  "ID374_outdoor_scanner_API.MessageStatus.Length"
  outdoor_scanner_API/11 -> Out Bus Element10/1  "ID374_outdoor_scanner_API.MessageStatus.Status"

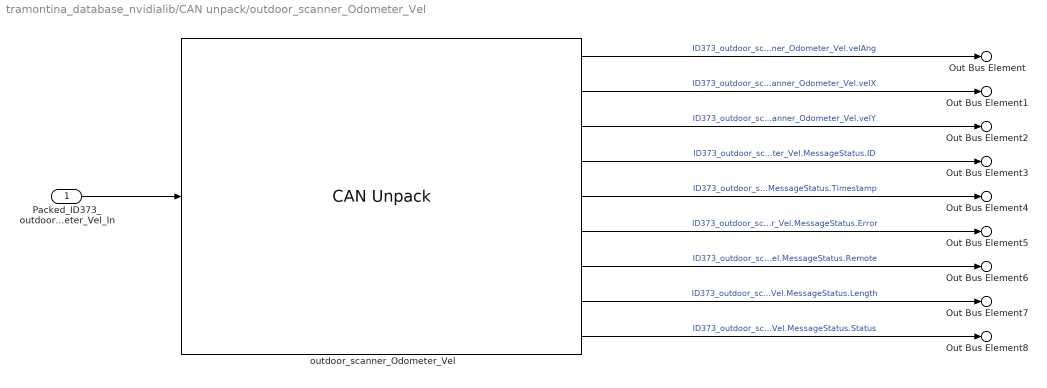
== system tramontina_database_nvidialib/CAN unpack/outdoor_scanner_Odometer_Vel ==
  Packed_ID373_outdoor_scanner_Odometer_Vel_In : Inport
  outdoor_scanner_Odometer_Vel : canmsglib/CAN Unpack  CANdbFile=C:\Users\matlab.cut\Desktop\AMR\canbus_files\tramontina_database_nvidia.dbc  MsgList=outdoor_scanner_Odometer_Vel  MsgName=outdoor_scanner_Odometer_Vel  MsgIDType=Standard (11-bit identifier)  MsgIdentifier=373  MsgLength=8  SignalInfo={'velAng','32','32','LE','single','Standard','0','1','0','-2147483648','-2147483648';'velX','0','16','LE','signed','Standard','0','1','0','-32768','32768';'velY','16','16','LE','signed','Standard','0','1','0','-32768','32768'}  IDPort=on  TimestampPort=on  ErrorPort=on  RemotePort=on  LengthPort=on  StatusPort=on  ApplyMinMax=off
  Out Bus Element : Outport  PortName=ID373_outdoor_scanner_Odometer_Vel  Element=velAng
  Out Bus Element1 : Outport  PortName=ID373_outdoor_scanner_Odometer_Vel  Element=velX
  Out Bus Element2 : Outport  PortName=ID373_outdoor_scanner_Odometer_Vel  Element=velY
  Out Bus Element3 : Outport  PortName=ID373_outdoor_scanner_Odometer_Vel  Element=MessageStatus.ID
  Out Bus Element4 : Outport  PortName=ID373_outdoor_scanner_Odometer_Vel  Element=MessageStatus.Timestamp
  Out Bus Element5 : Outport  PortName=ID373_outdoor_scanner_Odometer_Vel  Element=MessageStatus.Error
  Out Bus Element6 : Outport  PortName=ID373_outdoor_scanner_Odometer_Vel  Element=MessageStatus.Remote
  Out Bus Element7 : Outport  PortName=ID373_outdoor_scanner_Odometer_Vel  Element=MessageStatus.Length
  Out Bus Element8 : Outport  PortName=ID373_outdoor_scanner_Odometer_Vel  Element=MessageStatus.Status
  wires:
  Packed_ID373_outdoor_scanner_Odometer_Vel_In/1 -> outdoor_scanner_Odometer_Vel/1
  outdoor_scanner_Odometer_Vel/1 -> Out Bus Element/1  "ID373_outdoor_scanner_Odometer_Vel.velAng"
  outdoor_scanner_Odometer_Vel/2 -> Out Bus Element1/1  "ID373_outdoor_scanner_Odometer_Vel.velX"
  outdoor_scanner_Odometer_Vel/3 -> Out Bus Element2/1  "ID373_outdoor_scanner_Odometer_Vel.velY"
  outdoor_scanner_Odometer_Vel/4 -> Out Bus Element3/1  "ID373_outdoor_scanner_Odometer_Vel.MessageStatus.ID"
  outdoor_scanner_Odometer_Vel/5 -> Out Bus Element4/1  "ID373_outdoor_scanner_Odometer_Vel.MessageStatus.Timestamp"
  outdoor_scanner_Odometer_Vel/6 -> Out Bus Element5/1  "ID373_outdoor_scanner_Odometer_Vel.MessageStatus.Error"
  outdoor_scanner_Odometer_Vel/7 -> Out Bus Element6/1  "ID373_outdoor_scanner_Odometer_Vel.MessageStatus.Remote"
  outdoor_scanner_Odometer_Vel/8 -> Out Bus Element7/1  "ID373_outdoor_scanner_Odometer_Vel.MessageStatus.Length"
  outdoor_scanner_Odometer_Vel/9 -> Out Bus Element8/1  "ID373_outdoor_scanner_Odometer_Vel.MessageStatus.Status"

== system tramontina_database_nvidialib/CAN unpack/outdoor_scanner_PosX ==
  Packed_ID370_outdoor_scanner_PosX_In : Inport
  outdoor_scanner_PosX : canmsglib/CAN Unpack  CANdbFile=C:\Users\matlab.cut\Desktop\AMR\canbus_files\tramontina_database_nvidia.dbc  MsgList=outdoor_scanner_PosX  MsgName=outdoor_scanner_PosX  MsgIDType=Standard (11-bit identifier)  MsgIdentifier=370  MsgLength=8  SignalInfo={'X','0','64','LE','double','Standard','0','1','0','-9.2233720369e+18','9.2233720369e+18'}  IDPort=on  TimestampPort=on  ErrorPort=on  RemotePort=on  LengthPort=on  StatusPort=on  ApplyMinMax=off
  Out Bus Element : Outport  PortName=ID370_outdoor_scanner_PosX  Element=X
  Out Bus Element1 : Outport  PortName=ID370_outdoor_scanner_PosX  Element=MessageStatus.ID
  Out Bus Element2 : Outport  PortName=ID370_outdoor_scanner_PosX  Element=MessageStatus.Timestamp
  Out Bus Element3 : Outport  PortName=ID370_outdoor_scanner_PosX  Element=MessageStatus.Error
  Out Bus Element4 : Outport  PortName=ID370_outdoor_scanner_PosX  Element=MessageStatus.Remote
  Out Bus Element5 : Outport  PortName=ID370_outdoor_scanner_PosX  Element=MessageStatus.Length
  Out Bus Element6 : Outport  PortName=ID370_outdoor_scanner_PosX  Element=MessageStatus.Status
  wires:
  Packed_ID370_outdoor_scanner_PosX_In/1 -> outdoor_scanner_PosX/1
  outdoor_scanner_PosX/1 -> Out Bus Element/1  "ID370_outdoor_scanner_PosX.X"
  outdoor_scanner_PosX/2 -> Out Bus Element1/1  "ID370_outdoor_scanner_PosX.MessageStatus.ID"
  outdoor_scanner_PosX/3 -> Out Bus Element2/1  "ID370_outdoor_scanner_PosX.MessageStatus.Timestamp"
  outdoor_scanner_PosX/4 -> Out Bus Element3/1  "ID370_outdoor_scanner_PosX.MessageStatus.Error"
  outdoor_scanner_PosX/5 -> Out Bus Element4/1  "ID370_outdoor_scanner_PosX.MessageStatus.Remote"
  outdoor_scanner_PosX/6 -> Out Bus Element5/1  "ID370_outdoor_scanner_PosX.MessageStatus.Length"
  outdoor_scanner_PosX/7 -> Out Bus Element6/1  "ID370_outdoor_scanner_PosX.MessageStatus.Status"

== system tramontina_database_nvidialib/CAN unpack/outdoor_scanner_PosY ==
  Packed_ID371_outdoor_scanner_PosY_In : Inport
  outdoor_scanner_PosY : canmsglib/CAN Unpack  CANdbFile=C:\Users\matlab.cut\Desktop\AMR\canbus_files\tramontina_database_nvidia.dbc  MsgList=outdoor_scanner_PosY  MsgName=outdoor_scanner_PosY  MsgIDType=Standard (11-bit identifier)  MsgIdentifier=371  MsgLength=8  SignalInfo={'Y','0','64','LE','double','Standard','0','1','0','-9.2233720369e+18','9.2233720369e+18'}  IDPort=on  TimestampPort=on  ErrorPort=on  RemotePort=on  LengthPort=on  StatusPort=on  ApplyMinMax=off
  Out Bus Element : Outport  PortName=ID371_outdoor_scanner_PosY  Element=Y
  Out Bus Element1 : Outport  PortName=ID371_outdoor_scanner_PosY  Element=MessageStatus.ID
  Out Bus Element2 : Outport  PortName=ID371_outdoor_scanner_PosY  Element=MessageStatus.Timestamp
  Out Bus Element3 : Outport  PortName=ID371_outdoor_scanner_PosY  Element=MessageStatus.Error
  Out Bus Element4 : Outport  PortName=ID371_outdoor_scanner_PosY  Element=MessageStatus.Remote
  Out Bus Element5 : Outport  PortName=ID371_outdoor_scanner_PosY  Element=MessageStatus.Length
  Out Bus Element6 : Outport  PortName=ID371_outdoor_scanner_PosY  Element=MessageStatus.Status
  wires:
  Packed_ID371_outdoor_scanner_PosY_In/1 -> outdoor_scanner_PosY/1
  outdoor_scanner_PosY/1 -> Out Bus Element/1  "ID371_outdoor_scanner_PosY.Y"
  outdoor_scanner_PosY/2 -> Out Bus Element1/1  "ID371_outdoor_scanner_PosY.MessageStatus.ID"
  outdoor_scanner_PosY/3 -> Out Bus Element2/1  "ID371_outdoor_scanner_PosY.MessageStatus.Timestamp"
  outdoor_scanner_PosY/4 -> Out Bus Element3/1  "ID371_outdoor_scanner_PosY.MessageStatus.Error"
  outdoor_scanner_PosY/5 -> Out Bus Element4/1  "ID371_outdoor_scanner_PosY.MessageStatus.Remote"
  outdoor_scanner_PosY/6 -> Out Bus Element5/1  "ID371_outdoor_scanner_PosY.MessageStatus.Length"
  outdoor_scanner_PosY/7 -> Out Bus Element6/1  "ID371_outdoor_scanner_PosY.MessageStatus.Status"

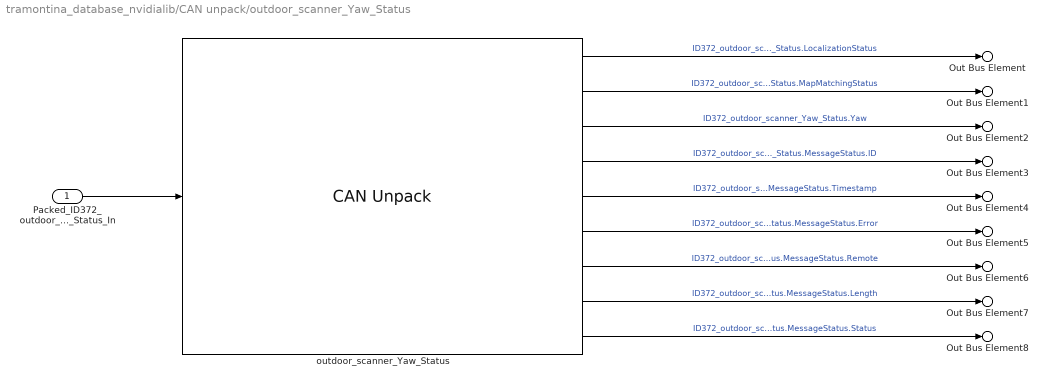
== system tramontina_database_nvidialib/CAN unpack/outdoor_scanner_Yaw_Status ==
  Packed_ID372_outdoor_scanner_Yaw_Status_In : Inport
  outdoor_scanner_Yaw_Status : canmsglib/CAN Unpack  CANdbFile=C:\Users\matlab.cut\Desktop\AMR\canbus_files\tramontina_database_nvidia.dbc  MsgList=outdoor_scanner_Yaw_Status  MsgName=outdoor_scanner_Yaw_Status  MsgIDType=Standard (11-bit identifier)  MsgIdentifier=372  MsgLength=6  SignalInfo={'LocalizationStatus','32','8','LE','unsigned','Standard','0','1','0','-Inf','Inf';'MapMatchingStatus','40','8','LE','unsigned','Standard','0','1','0','-Inf','Inf';'Yaw','0','32','LE','signed','Standard','0','1','0','-180000','180000'}  IDPort=on  TimestampPort=on  ErrorPort=on  RemotePort=on  LengthPort=on  StatusPort=on  ApplyMinMax=off
  Out Bus Element : Outport  PortName=ID372_outdoor_scanner_Yaw_Status  Element=LocalizationStatus
  Out Bus Element1 : Outport  PortName=ID372_outdoor_scanner_Yaw_Status  Element=MapMatchingStatus
  Out Bus Element2 : Outport  PortName=ID372_outdoor_scanner_Yaw_Status  Element=Yaw
  Out Bus Element3 : Outport  PortName=ID372_outdoor_scanner_Yaw_Status  Element=MessageStatus.ID
  Out Bus Element4 : Outport  PortName=ID372_outdoor_scanner_Yaw_Status  Element=MessageStatus.Timestamp
  Out Bus Element5 : Outport  PortName=ID372_outdoor_scanner_Yaw_Status  Element=MessageStatus.Error
  Out Bus Element6 : Outport  PortName=ID372_outdoor_scanner_Yaw_Status  Element=MessageStatus.Remote
  Out Bus Element7 : Outport  PortName=ID372_outdoor_scanner_Yaw_Status  Element=MessageStatus.Length
  Out Bus Element8 : Outport  PortName=ID372_outdoor_scanner_Yaw_Status  Element=MessageStatus.Status
  wires:
  Packed_ID372_outdoor_scanner_Yaw_Status_In/1 -> outdoor_scanner_Yaw_Status/1
  outdoor_scanner_Yaw_Status/1 -> Out Bus Element/1  "ID372_outdoor_scanner_Yaw_Status.LocalizationStatus"
  outdoor_scanner_Yaw_Status/2 -> Out Bus Element1/1  "ID372_outdoor_scanner_Yaw_Status.MapMatchingStatus"
  outdoor_scanner_Yaw_Status/3 -> Out Bus Element2/1  "ID372_outdoor_scanner_Yaw_Status.Yaw"
  outdoor_scanner_Yaw_Status/4 -> Out Bus Element3/1  "ID372_outdoor_scanner_Yaw_Status.MessageStatus.ID"
  outdoor_scanner_Yaw_Status/5 -> Out Bus Element4/1  "ID372_outdoor_scanner_Yaw_Status.MessageStatus.Timestamp"
  outdoor_scanner_Yaw_Status/6 -> Out Bus Element5/1  "ID372_outdoor_scanner_Yaw_Status.MessageStatus.Error"
  outdoor_scanner_Yaw_Status/7 -> Out Bus Element6/1  "ID372_outdoor_scanner_Yaw_Status.MessageStatus.Remote"
  outdoor_scanner_Yaw_Status/8 -> Out Bus Element7/1  "ID372_outdoor_scanner_Yaw_Status.MessageStatus.Length"
  outdoor_scanner_Yaw_Status/9 -> Out Bus Element8/1  "ID372_outdoor_scanner_Yaw_Status.MessageStatus.Status"

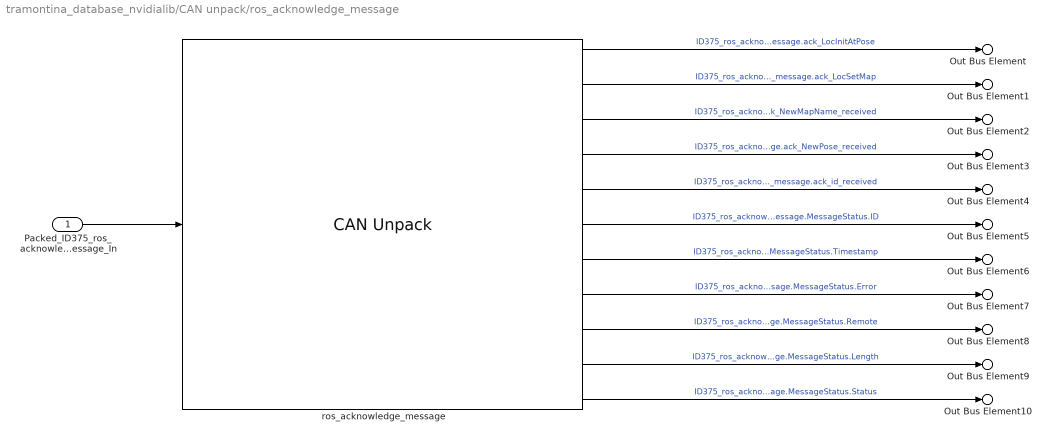
== system tramontina_database_nvidialib/CAN unpack/ros_acknowledge_message ==
  Packed_ID375_ros_acknowledge_message_In : Inport
  ros_acknowledge_message : canmsglib/CAN Unpack  CANdbFile=C:\Users\matlab.cut\Desktop\AMR\canbus_files\tramontina_database_nvidia.dbc  MsgList=ros_acknowledge_message  MsgName=ros_acknowledge_message  MsgIDType=Standard (11-bit identifier)  MsgIdentifier=375  MsgLength=1  SignalInfo={'ack_LocInitAtPose','3','1','LE','unsigned','Standard','0','1','0','-Inf','Inf';'ack_LocSetMap','4','1','LE','unsigned','Standard','0','1','0','-Inf','Inf';'ack_NewMapName_received','1','1','LE','unsigned','Standard','0','1','0','-Inf','Inf';'ack_NewPose_received','2','1','LE','unsigned','Standard','0','1','0','-Inf','Inf';'ack_id_received','0','1','LE','unsigned','Standard','0','1','0','0','1'}  IDPort=on  TimestampPort=on  ErrorPort=on  RemotePort=on  LengthPort=on  StatusPort=on  ApplyMinMax=off
  Out Bus Element : Outport  PortName=ID375_ros_acknowledge_message  Element=ack_LocInitAtPose
  Out Bus Element1 : Outport  PortName=ID375_ros_acknowledge_message  Element=ack_LocSetMap
  Out Bus Element2 : Outport  PortName=ID375_ros_acknowledge_message  Element=ack_NewMapName_received
  Out Bus Element3 : Outport  PortName=ID375_ros_acknowledge_message  Element=ack_NewPose_received
  Out Bus Element4 : Outport  PortName=ID375_ros_acknowledge_message  Element=ack_id_received
  Out Bus Element5 : Outport  PortName=ID375_ros_acknowledge_message  Element=MessageStatus.ID
  Out Bus Element6 : Outport  PortName=ID375_ros_acknowledge_message  Element=MessageStatus.Timestamp
  Out Bus Element7 : Outport  PortName=ID375_ros_acknowledge_message  Element=MessageStatus.Error
  Out Bus Element8 : Outport  PortName=ID375_ros_acknowledge_message  Element=MessageStatus.Remote
  Out Bus Element9 : Outport  PortName=ID375_ros_acknowledge_message  Element=MessageStatus.Length
  Out Bus Element10 : Outport  PortName=ID375_ros_acknowledge_message  Element=MessageStatus.Status
  wires:
  Packed_ID375_ros_acknowledge_message_In/1 -> ros_acknowledge_message/1
  ros_acknowledge_message/1 -> Out Bus Element/1  "ID375_ros_acknowledge_message.ack_LocInitAtPose"
  ros_acknowledge_message/2 -> Out Bus Element1/1  "ID375_ros_acknowledge_message.ack_LocSetMap"
  ros_acknowledge_message/3 -> Out Bus Element2/1  "ID375_ros_acknowledge_message.ack_NewMapName_received"
  ros_acknowledge_message/4 -> Out Bus Element3/1  "ID375_ros_acknowledge_message.ack_NewPose_received"
  ros_acknowledge_message/5 -> Out Bus Element4/1  "ID375_ros_acknowledge_message.ack_id_received"
  ros_acknowledge_message/6 -> Out Bus Element5/1  "ID375_ros_acknowledge_message.MessageStatus.ID"
  ros_acknowledge_message/7 -> Out Bus Element6/1  "ID375_ros_acknowledge_message.MessageStatus.Timestamp"
  ros_acknowledge_message/8 -> Out Bus Element7/1  "ID375_ros_acknowledge_message.MessageStatus.Error"
  ros_acknowledge_message/9 -> Out Bus Element8/1  "ID375_ros_acknowledge_message.MessageStatus.Remote"
  ros_acknowledge_message/10 -> Out Bus Element9/1  "ID375_ros_acknowledge_message.MessageStatus.Length"
  ros_acknowledge_message/11 -> Out Bus Element10/1  "ID375_ros_acknowledge_message.MessageStatus.Status"
